simulink model "Problem2"  (R2020a)
settings: Solver=FixedStepDiscrete  StartTime=0.0  StopTime=150  FixedStep=0.1  RelTol=1e-3  EnableMultiTasking=on
undefined symbols (not defined in the file): DiscIntNeverNeededParam
libraries: simulink x1
settings Model: Creator=aishw  LastModifiedBy=aishw
settings DataIOCC: LimitDataPoints=on  SaveFormat=Array  ReturnWorkspaceOutputs=off

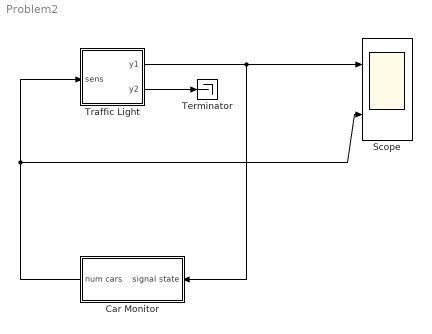
== system Problem2 ==
  Car Monitor : Subsystem
  Scope : Scope  NumInputPorts=2
  Terminator : Terminator
  Traffic Light : Stateflow chart  TreatAsAtomicUnit=on
  wires:
  Car Monitor/1(num cars) -> Traffic Light/1(sens), Scope/2
  Traffic Light/2(y2) -> Terminator/1
  Traffic Light/1(y1) -> Car Monitor/1(signal state), Scope/1

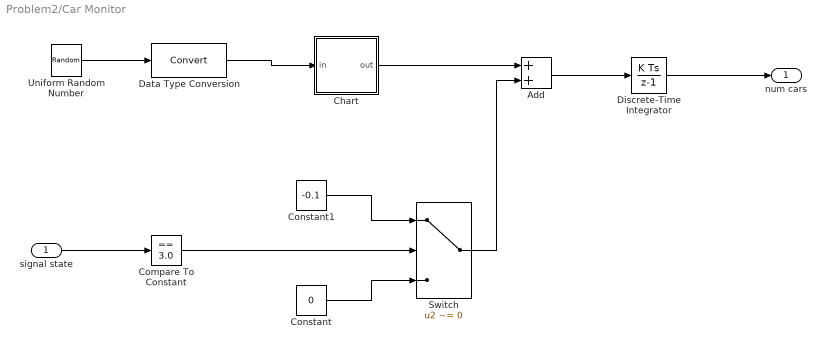
== system Problem2/Car Monitor ==
  signal state : Inport
  Add : Sum
  Chart : Stateflow chart  TreatAsAtomicUnit=on
  Compare To Constant : simulink/Logic and Bit Operations/Compare To Constant  relop===  const=3.0  OutDataTypeStr=boolean
  Constant : Constant  Value=0
  Constant1 : Constant  Value=-0.1
  Data Type Conversion : DataTypeConversion
  Discrete-Time Integrator : DiscreteIntegrator  SampleTime=-1  LimitOutput=on  LowerSaturationLimit=0  ICPrevOutput=DiscIntNeverNeededParam  ICPrevScaledInput=DiscIntNeverNeededParam
  Switch : Switch  Criteria=u2 ~= 0
  Uniform Random Number : UniformRandomNumber  Minimum=0  Maximum=100  Seed=177836  SampleTime=0
  num cars : Outport
  wires:
  Uniform Random Number/1 -> Data Type Conversion/1
  Data Type Conversion/1 -> Chart/1(in)
  Chart/1(out) -> Add/1
  signal state/1 -> Compare To Constant/1
  Compare To Constant/1 -> Switch/2
  Constant1/1 -> Switch/1
  Constant/1 -> Switch/3
  Switch/1 -> Add/2
  Add/1 -> Discrete-Time Integrator/1
  Discrete-Time Integrator/1 -> num cars/1

== stateflow chart Problem2/Car Monitor/Chart ==
  (default) -> (junction 6) : {out = in > 98;}
  data: in input; out output

== stateflow chart Problem2/Traffic Light ==
  settings: stateMachineType=MOORE_MACHINE  initializeOutput=1
  state Stop
    y1 = RED;
    y2 = GREEN;
  state StopforTraffic
    y1 = RED;
    y2 = GREEN;
  state StoptoGO
    y1 = RED;
    y2  = YELLOW;
  state GotoStop
    y1 = YELLOW;
    y2 = RED;
  state Go
    y1 = GREEN;
    y2 = RED;
  (default) -> Stop
  Stop -> StopforTraffic : after(20,tick)
  StopforTraffic -> StoptoGO : [sens]
  GotoStop -> Stop : after(3,tick)
  StoptoGO -> Go : after(3,tick)
  Go -> GotoStop : after(10,tick)
  data: y1 output; sens input; y2 output; GREEN constant double =3; RED constant double =1; YELLOW constant double =2
